simulink model "truck_pid"  (R2024a)
settings: Solver=ode45  StartTime=0.0  StopTime=100.0  RelTol=1e-1
libraries: truck_lib x1
settings Model: Creator=adriaeik  LastModifiedBy=eikel

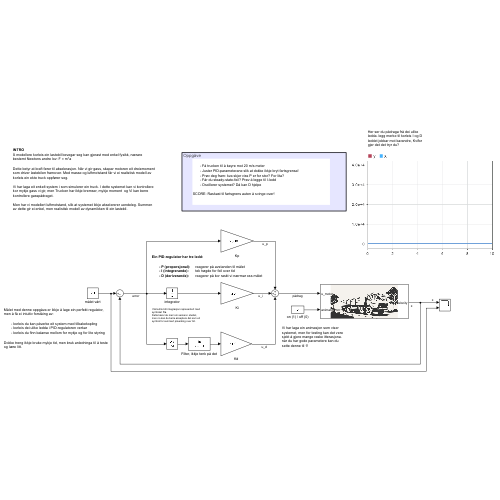
[thumbnail: Simulink's stored preview of the top-level diagram]
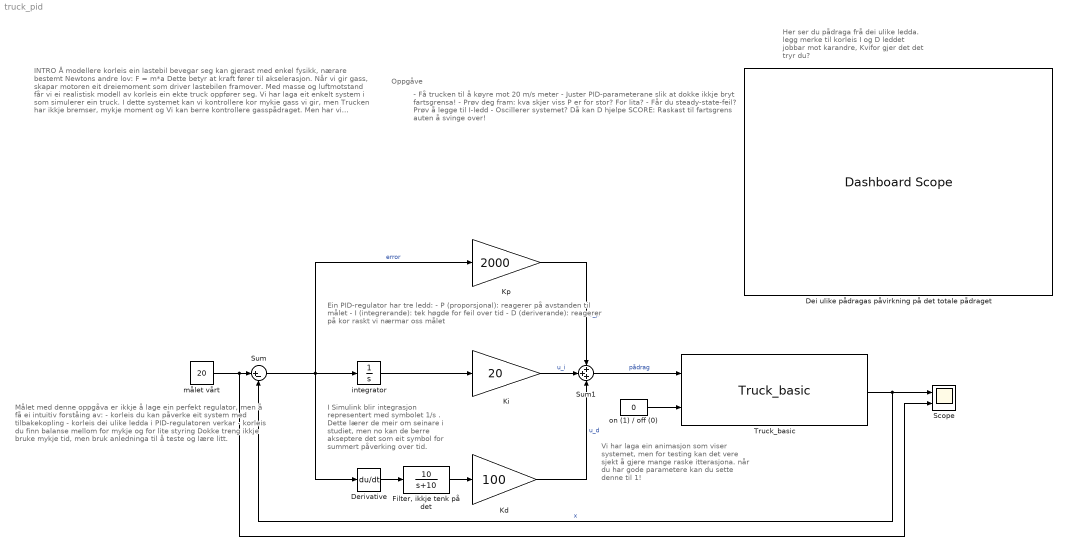
== system truck_pid ==
  note: Vi har laga ein animasjon som viser systemet, men for testing kan det vere sjekt å gjere mange raske itterasjona. når du har gode parametere kan du sette denne til 1!
  note: Her ser du pådraga frå dei ulike ledda. legg merke til korleis I og D leddet jobbar mot karandre, Kvifor gjer det det tryr du?
  note: Oppgåve
  note: - Få trucken til å køyre mot 20 m/s meter
      | 	- Juster PID-parameterane slik at dokke ikkje bryt fartsgrensa!
      | 	- Prøv deg fram: kva skjer viss P er for stor? For lita?
      | 	- Får du steady-state-feil? Prøv å legge til I-ledd
      | 	- Oscillerer systemet? Då kan D hjelpe
      |
      | SCORE: Raskast til fartsgrens auten å svinge over!
  note: Målet med denne oppgåva er ikkje å lage ein perfekt regulator, men å få ei intuitiv forståing av:
      |
      | 	- korleis du kan påverke eit system med tilbakekopling
      | 	- korleis dei ulike ledda i PID-regulatoren verkar
      | 	- korleis du finn balanse mellom for mykje og for lite styring
      |
      | Dokke treng ikkje bruke mykje tid, men bruk anledninga til å teste og lære litt.
  note: Ein PID-regulator har tre ledd:
      |
      | - P (proporsjonal): reagerer på avstanden til målet
      | - I (integrerande): tek høgde for feil over tid
      | - D (deriverande): reagerer på kor raskt vi nærmar oss målet
  note: INTRO
      | Å modellere korleis ein lastebil bevegar seg kan gjerast med enkel fysikk, nærare bestemt Newtons andre lov: F = m*a
      |
      | Dette betyr at kraft fører til akselerasjon. Når vi gir gass, skapar motoren eit dreiemoment som driver lastebilen framover. Med masse og luftmotstand får vi ei realistisk modell av korleis ein ekte truck oppfører seg.
      |
      | Vi har laga eit enkelt system i som simulerer ein truck. I dette systemet kan vi kontrollere kor mykje gass vi gir, men Trucken har ikkje bremser, mykje moment og Vi kan berre kontrollere gasspådraget.
      |
      | Men har vi modellert luftmotstand, slik at systemet ikkje akselererer uendeleg. Summen av dette gir ei enkel, men realistisk modell av dynamikken til ein lastebil.
  note: I Simulink blir integrasjon representert med symbolet 1/s .
      | Dette lærer de meir om seinare i studiet, men no kan de berre akseptere det som eit symbol for summert påverking over tid.
  Dei ulike pådragas påvirkning på det totale pådraget : DashboardScope
  Derivative : Derivative
  "Filter, ikkje tenk på det" : TransferFcn  Numerator=[10]  Denominator=[1 10]
  Kd : Gain  Gain=100
  Ki : Gain  Gain=20
  Kp : Gain  Gain=2000
  Scope : Scope  NumInputPorts=2
  Sum : Sum  Inputs=|+-
  Sum1 : Sum  Inputs=+++
  Truck_basic : truck_lib/Truck_basic  SystemSampleTime=-1  VariantActivationTime=update diagram  AllowFlexibleInterface=on  Latency=0  AutoFrameSizeCalculation=off
  integrator : Integrator
  målet vårt : Constant  Value=20
  on (1) / off (0) : Constant  Value=0
  wires:
  Sum1/1 -> Truck_basic/1  "pådrag"
  Truck_basic/1 -> Scope/1, Sum/2  "x"
  Sum/1 -> Kp/1, Derivative/1, integrator/1  "error"
  målet vårt/1 -> Scope/2, Sum/1
  Derivative/1 -> "Filter, ikkje tenk på det"/1
  integrator/1 -> Ki/1
  "Filter, ikkje tenk på det"/1 -> Kd/1
  Ki/1 -> Sum1/2  "u_i"
  Kp/1 -> Sum1/1  "u_p"
  Kd/1 -> Sum1/3  "u_d"
  on (1) / off (0)/1 -> Truck_basic/2
